simulink model "modello_fisico"  (R2024b)
settings: Solver=VariableStepAuto  StartTime=0.0  StopTime=50  RelTol=1e-6
values from neighbouring files (symbols this model uses):
  alpha = l*m*g    (= 0.623916)    [Inizializzazione_modello_fisico.m]
  Cb = 1.02e-3    (= 0.00102)    [Inizializzazione_modello_fisico.m]    (also in cubo1D_calcolo.m)
  Cw = 0.05e-3    (= 5e-05)    [Inizializzazione_modello_fisico.m]    (also in cubo1D_calcolo.m)
  Ib = 0.57e-3    (= 0.00057)    [Inizializzazione_modello_fisico.m]    (also in cubo1D_calcolo.m = 0.00334)
  Iw = 3.34e-3    (= 0.00334)    [Inizializzazione_modello_fisico.m]    (also in cubo1D_calcolo.m = 0.00057)
settings Model: Creator=Hp  LastModifiedBy=Hp

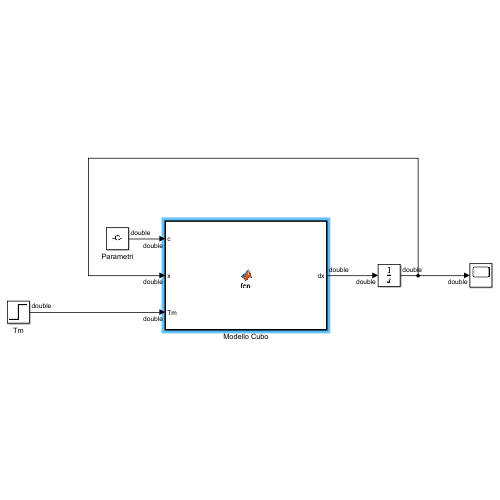
[thumbnail: Simulink's stored preview of the top-level diagram]
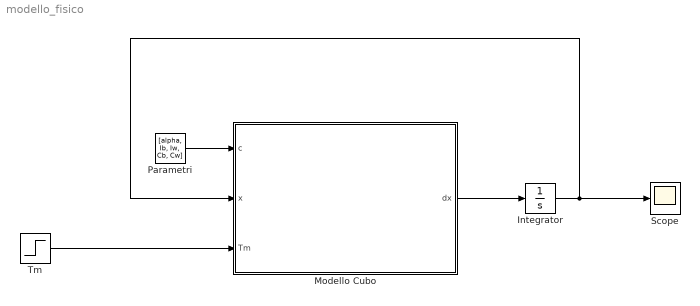
== system modello_fisico ==
  Integrator : Integrator
  Modello Cubo : MATLAB Function  TreatAsAtomicUnit=on
  Parametri : Constant  Value=[alpha, Ib, Iw, Cb, Cw]
  Scope : Scope
  Tm : Step  Time=3  After=5  SampleTime=0
  wires:
  Modello Cubo/1(dx) -> Integrator/1
  Integrator/1 -> Scope/1, Modello Cubo/2(x)
  Parametri/1 -> Modello Cubo/1(c)
  Tm/1 -> Modello Cubo/3(Tm)

== matlab function modello_fisico/Modello Cubo ==
  data: c input double size=[5 1]; dx output double size=[1 3]; x input double size=[1 3]; Tm input
function dx = fcn(c, x, Tm)
%Vettore di stato x(theta_b, dtheta_b, dtheta_w)
theta_b=x(1);
dtheta_b=x(2);
dtheta_w=x(3);

%Vettore delle costanti
alpha=c(1);
Ib=c(2);
Iw=c(3);
Cb=c(4);
Cw=c(5);

%Impostiamo i 2 denominatori e il seno(theta_b)
den1=Ib;
den2=Ib*Iw;
st=sin(theta_b);

%Equazioni di Eulero Lagrange
ddtheta_b=(alpha*st-Tm+Cw*dtheta_w-Cb*dtheta_b)/den1;
ddtheta_w=(Tm*(Ib+Iw)-Cw*dtheta_w*(Ib+Iw)-alpha*st*Iw+Cb*dtheta_b*Iw)/den2;

dx=[dtheta_b, ddtheta_b, ddtheta_w]; %out
